simulink model "sldemo_tonegen_fixpt"  (Simulink 7.6)
settings: Solver=FixedStepDiscrete  SolverMode=SingleTasking  StartTime=0  StopTime=30  FixedStep=1/256  RelTol=1e-3
StartFcn:
  | if exist('tonegenfxpt_ploth')
  |   if ishghandle(tonegenfxpt_ploth,'figure'), close(tonegenfxpt_ploth); end
  |   clear tonegenfxpt_ploth
  | end
StopFcn:
  | if exist('tonegenOut')
  |  if ~isnumeric(tonegenOut)
  |   tonegenfxpt_ploth = figure;
  |   subplot(4,1,1), plot(tonegenOut.time, tonegenOut.signals(1).values); grid
  |   title('Difference between direct look-up and reference signal');
  |   subplot(4,1,2), plot(tonegenOut.time, tonegenOut.signals(2).values); grid
  |   title('Difference between interpolated look-up and reference signal');
  |   subplot(4,1,3), plot(tonegenOut.time, tonegenOut.signals(3).values); grid
  |   title('Difference between CORDIC sine and reference signal');
  |   subplot(4,1,4), plot(tonegenOut.time, tonegenOut.signals(4).values); grid
  |   title('Difference between time based sin() and reference signal');
  | end
  | end
libraries: simulink x2
Description:
  | Generating Sine Waves with Floating Point and Fixed Point Data
  | 
  | This model lets you compare a variety of techniques available in
  | Simulink for generating sine waves.Simulink includes a sine wave source
  | block with continuous and discrete modes, plus fixed point sine and
  | cosine function blocks that implement the function approximation with
  | a linearly interpolated lookup table that exploits the quarter wave
  | symmetry of sine and cosine.  The model also compares fixed point sine
  | CORDIC approximation from Trigonometric Function block with the reference
  | signal.
CloseFcn:
  | if exist('tonegenfxpt_ploth')
  |   if ishghandle(tonegenfxpt_ploth,'figure'), close(tonegenfxpt_ploth); end
  |   clear tonegenfxpt_ploth
  |   if exist('tonegenOut'), clear tonegenOut; end
  | end
settings Model: Creator=The MathWorks Inc.  ExtModeAutoUpdateStatusClock=off
settings DataIOCC: LimitDataPoints=off  SaveFormat=StructureWithTime  SaveTime=off  OutputSaveName=tonegenOut  SignalLoggingName=sigsOut
settings OptimizationCC: InlineInvariantSignals=on  InitFltsAndDblsToZero=on  BufferReusableBoundary=off
settings DebuggingCC: SaveWithParameterizedLinksMsg=none  CheckExecutionContextPreStartOutputMsg=on  CheckExecutionContextRuntimeOutputMsg=on  SignalResolutionControl=TryResolveAllWithWarning  SolverPrmCheckMsg=none  MultiTaskDSMMsg=warning  MultiTaskCondExecSysMsg=none  IntegerOverflowMsg=none  ParameterPrecisionLossMsg=none  BusObjectLabelMismatch=none
settings HardwareCC: TargetUnknown=on
settings RTWCC: IncludeERTFirstTime=on
settings CodeAppCC: CustomSymbolStrFcn=$F$N$M
settings GRTTargetCC: TargetFcnLib=ansi_tfl_tmw.mat

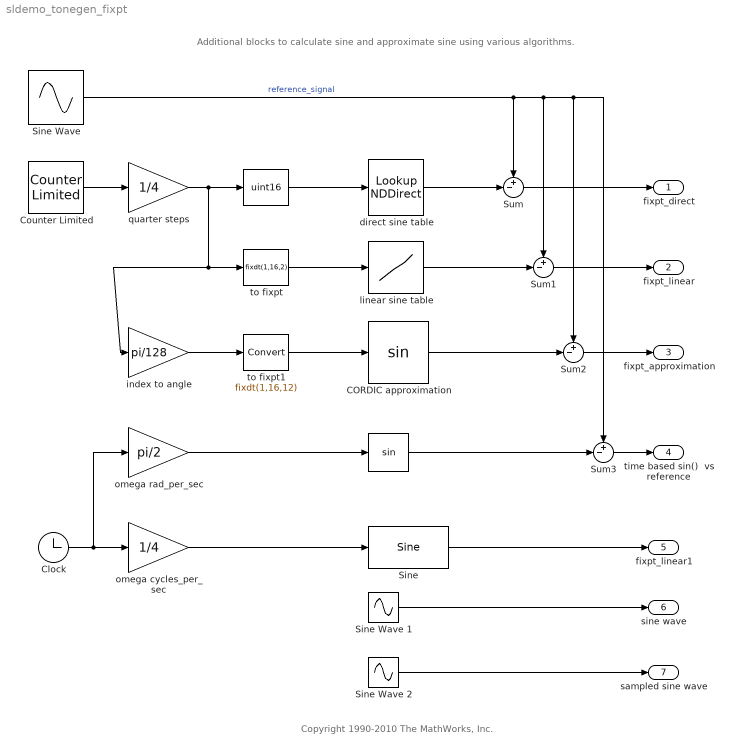
== system sldemo_tonegen_fixpt ==
  note: Additional blocks to calculate sine and
      | approximate sine using various algorithms.
  note: Copyright 1990-2010 The MathWorks, Inc.
  "  " : Trigonometry  NumberOfIterations=15
  "      " : DataTypeConversion  OutDataTypeStr=uint16
  CORDIC approximation : Trigonometry  ApproximationMethod=CORDIC  NumberOfIterations=15
  Clock : Clock
      settings: Decimation=10
  Counter Limited : simulink/Sources/Counter Limited  SystemSampleTime=-1  uplimit=1023  tsamp=-1
  Sine : simulink/Lookup Tables/Sine  SystemSampleTime=-1  Formula=sin(2*pi*u)  NumDataPoints=(2^5)+1  OutputWordLength=16
  Sine Wave : Sin  SineType=Sample based  Frequency=pi/2  Samples=1024  SampleTime=0.00390625
  Sine Wave 1 : Sin  SampleTime=0
  Sine Wave 2 : Sin  SineType=Sample based  Frequency=pi/2  SampleTime=1/256
  Sum{,1..3} (4 alike) : Sum  Inputs=+-|
  direct sine table : LookupNDDirect  NumberOfTableDimensions=1  Table=sin( 2*pi * (0:255)/256)'  TableDataTypeStr=fixdt(1,16,14)
  index to angle : Gain  Gain=pi/128  OutDataTypeStr=float('double')
  linear sine table : Lookup_n-D  NumberOfTableDimensions=1  BreakpointsForDimension1=[0:256]  IndexSearchMethod=Linear search  BeginIndexSearchUsingPreviousIndexResult=on  Table=sin( 2*pi * (0:256)/256 )'  ExtrapMethod=None - Clip  ActionForOutOfRangeInput=Warning  OutDataTypeStr=fixdt(1,16,14)  InputSameDT=on
  omega cycles_per_sec : Gain  Gain=1/4
  omega rad_per_sec : Gain  Gain=pi/2
  quarter steps : Gain  Gain=1/4  OutDataTypeStr=float('double')
  "to fixpt " : DataTypeConversion  OutDataTypeStr=fixdt(1,16,2)
  to fixpt1 : DataTypeConversion  OutDataTypeStr=fixdt(1,16,12)
  fixpt_direct : Outport
  fixpt_linear : Outport  Port=2
  fixpt_approximation : Outport  Port=3
  time based sin()  vs reference : Outport  Port=4
  fixpt_linear1 : Outport  Port=5
  sine wave : Outport  Port=6
  sampled sine wave : Outport  Port=7
  wires:
  Counter Limited/1 -> quarter steps/1
  quarter steps/1 -> index to angle/1, "to fixpt "/1, "      "/1
  Sine Wave/1 -> Sum2/1, Sum3/1, Sum1/1, Sum/1  "reference_signal"
  direct sine table/1 -> Sum/2
  linear sine table/1 -> Sum1/2
  Sum/1 -> fixpt_direct/1
  Sum1/1 -> fixpt_linear/1
  Sine/1 -> fixpt_linear1/1
  Clock/1 -> omega cycles_per_sec/1, omega rad_per_sec/1
  omega cycles_per_sec/1 -> Sine/1
  Sine Wave 1/1 -> sine wave/1
  Sine Wave 2/1 -> sampled sine wave/1
  Sum2/1 -> fixpt_approximation/1
  CORDIC approximation/1 -> Sum2/2
  index to angle/1 -> to fixpt1/1
  to fixpt1/1 -> CORDIC approximation/1
  "  "/1 -> Sum3/2
  Sum3/1 -> time based sin()  vs reference/1
  omega rad_per_sec/1 -> "  "/1
  "to fixpt "/1 -> linear sine table/1
  "      "/1 -> direct sine table/1
